simulink model "SiL"  (R2021a)
settings: Solver=VariableStepAuto  StartTime=0.0  StopTime=20  RelTol=1e-3
model workspace: external: MATLAB File C:\Users\Adam\OneDrive\Desktop\M.Sc_LRT\4.sem\session2\Stage\sim\InitMain.m (data not in the file)
values from neighbouring files (symbols this model uses):
  A_mpc = blkdiag([1 dt 0;0 1 dt;0 0 1],[1 dt 0;0 1 dt;0 0 1],[1 dt 0;0 1 dt;0 0 1])    [InitMain.m]    (also in init.m)
  B_mpc = zeros(9,3)    [InitMain.m]    (also in init.m)
  C_mpc = [1 zeros(1,8);0 0 0 1 zeros(1,5); zeros(1,6) 1 0 0 ... (first row only)    [InitMain.m]    (also in init.m)
  D_mpc = zeros(9,3)    [InitMain.m]    (also in init.m)
  dt = 0.01    [InitMain.m]    (also in init.m)
  g0 = 9.81    [InitMain.m]    (also in init.m)
  Ib = diag([0.035 0.046 0.0977])    [InitMain.m]    (also in init.m)
  K1 = Ka(:,1:12)    [InitMain.m]    (also in init.m)
  Ki = -Ka(:,13:16)    [InitMain.m]    (also in init.m)
  M = 1.5    [InitMain.m]    (also in init.m)
  wait = 5    [InitMain.m]    (also in init.m)
undefined symbols (not defined in the file or in its folder): C, Discrete, K_omega, k_omega, Kd_x, Kd_y, Kd_z, Ki_x, Ki_y, Ki_z, Kp_x, Kp_y, Kp_z, Kq_xy, Kq_z, kr, kv, kx, Time
libraries: sharedutil x7, vrlib x5, aerolibutil x3, sharedtransform x2, shared6dof x1, ctrlSharedLib x1, mpclib x1, drivingscenarioandsensors x1
settings Model: Creator=Adam  LastModifiedBy=Adam
settings SolverCC: ZeroCrossAlgorithm=Adaptive
settings DebuggingCC: MaskedZcDiagnostic=none  IgnoredZcDiagnostic=none  UnderSpecifiedDimensionMsg=warning

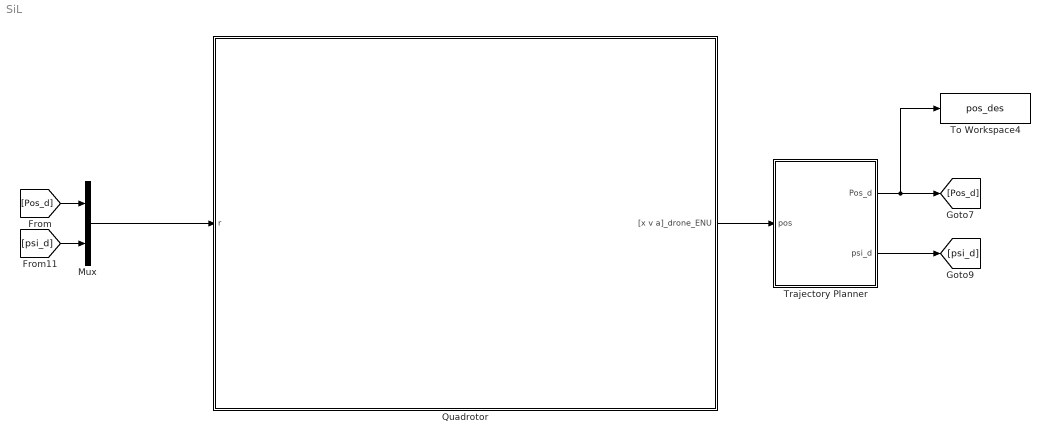
== system SiL ==
  Mux : Mux  Inputs=2
  Quadrotor : Subsystem
      mask Display: image('R.jpg'); % Use "Edit Image" on toolstrip to change.
  To Workspace4 : ToWorkspace  VariableName=pos_des  SaveFormat=Timeseries  SampleTime=-1
  Trajectory Planner : Subsystem
  wires:
  Trajectory Planner/1(Pos_d) -> To Workspace4/1, [Pos_d]
  Trajectory Planner/2(psi_d) -> [psi_d]
  [psi_d] -> Mux/2
  Mux/1 -> Quadrotor/1(r)
  [Pos_d] -> Mux/1
  Quadrotor/1("[x v a]_drone_ENU") -> Trajectory Planner/1(pos)

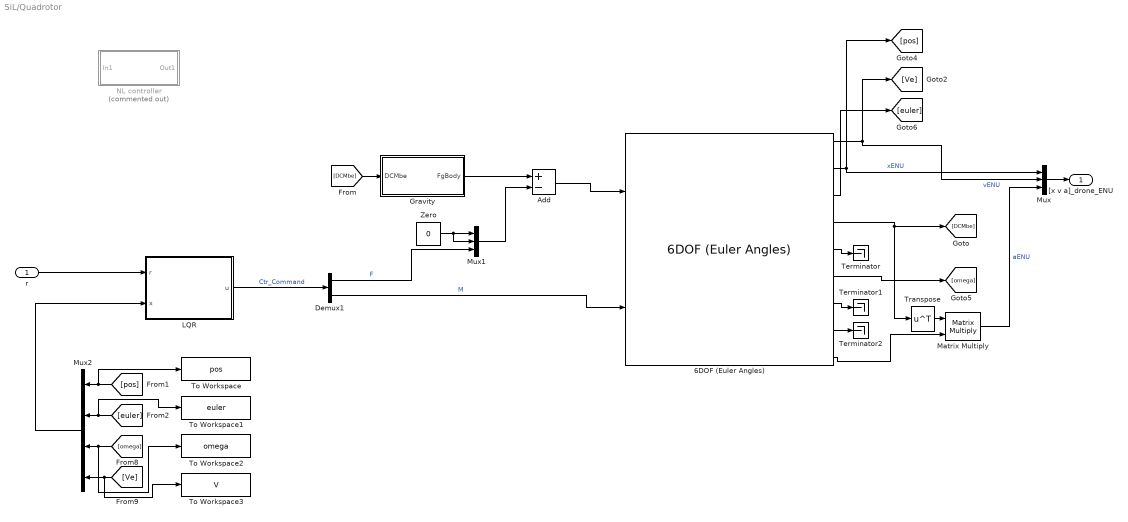
== system SiL/Quadrotor ==
  r : Inport
  6DOF (Euler Angles) : shared6dof/6DOF (Euler Angles)  units=Metric (MKS)  mtype=Fixed  rep=Euler Angles  xme_0=[0 0 0]  Vm_0=[0 0 0]  eul_0=[0 0 0]  pm_0=[0 0 0]  mass_0=M  mass_e=0.5  mass_f=2.0  inertia=Ib  inertia_e=eye(3)  inertia_f=2*eye(3)  k_quat=1.0  vre_flag=on  abi_flag=on  aMode=0  xme_statename='Xe'  Vm_statename='Ve'  eul_statename='Euler'  quat_statename=''  pm_statename='Omega'  mass_statename=''
      settings: SourceProductBaseCode=AE,PW,DR,MT,UV,VE
  Add : Sum  Inputs=+-
  Demux1 : Demux  Outputs=2
  "Gravity " : Subsystem
  LQR : Subsystem
  Matrix Multiply : Product  Multiplication=Matrix(*)
  Mux : Mux  Inputs=3
  Mux1 : Mux  Inputs=3
  Mux2 : Mux
  NL controller : Subsystem  Commented=on
  Terminator : Terminator
  Terminator1 : Terminator
  Terminator2 : Terminator
  To Workspace : ToWorkspace  VariableName=pos  SaveFormat=Timeseries  SampleTime=-1
  To Workspace1 : ToWorkspace  VariableName=euler  SaveFormat=Timeseries  SampleTime=-1
  To Workspace2 : ToWorkspace  VariableName=omega  SaveFormat=Timeseries  SampleTime=-1
  To Workspace3 : ToWorkspace  VariableName=V  SaveFormat=Timeseries  SampleTime=-1
  Transpose : Math  Operator=transpose  SaturateOnIntegerOverflow=on
  Zero : Constant  Value=0  OutDataTypeStr=Inherit: Inherit via back propagation
  "[x v a]_drone_ENU" : Outport
  wires:
  6DOF (Euler Angles)/7 -> Terminator1/1
  "Gravity "/1(FgBody) -> Add/1
  Add/1 -> 6DOF (Euler Angles)/1
  [DCMbe] -> "Gravity "/1(DCMbe)
  6DOF (Euler Angles)/1 -> Mux/2, [Ve]  "vENU"
  6DOF (Euler Angles)/2 -> Mux/1, [pos]  "xENU"
  6DOF (Euler Angles)/3 -> [euler]
  6DOF (Euler Angles)/6 -> [omega]
  6DOF (Euler Angles)/4 -> Transpose/1, [DCMbe]
  Zero/1 -> Mux1/2, Mux1/1
  Mux1/1 -> Add/2
  Demux1/1 -> Mux1/3  "F"
  Demux1/2 -> 6DOF (Euler Angles)/2  "M"
  Mux2/1 -> LQR/2(x)
  [pos] -> To Workspace/1, Mux2/1
  [euler] -> To Workspace1/1, Mux2/2
  LQR/1(u) -> Demux1/1  "Ctr_Command"
  [omega] -> To Workspace2/1, Mux2/3
  [Ve] -> Mux2/4, To Workspace3/1
  r/1 -> LQR/1(r)
  6DOF (Euler Angles)/5 -> Terminator/1
  Transpose/1 -> Matrix Multiply/1
  Matrix Multiply/1 -> Mux/3  "aENU"
  Mux/1 -> "[x v a]_drone_ENU"/1
  6DOF (Euler Angles)/9 -> Matrix Multiply/2
  6DOF (Euler Angles)/8 -> Terminator2/1

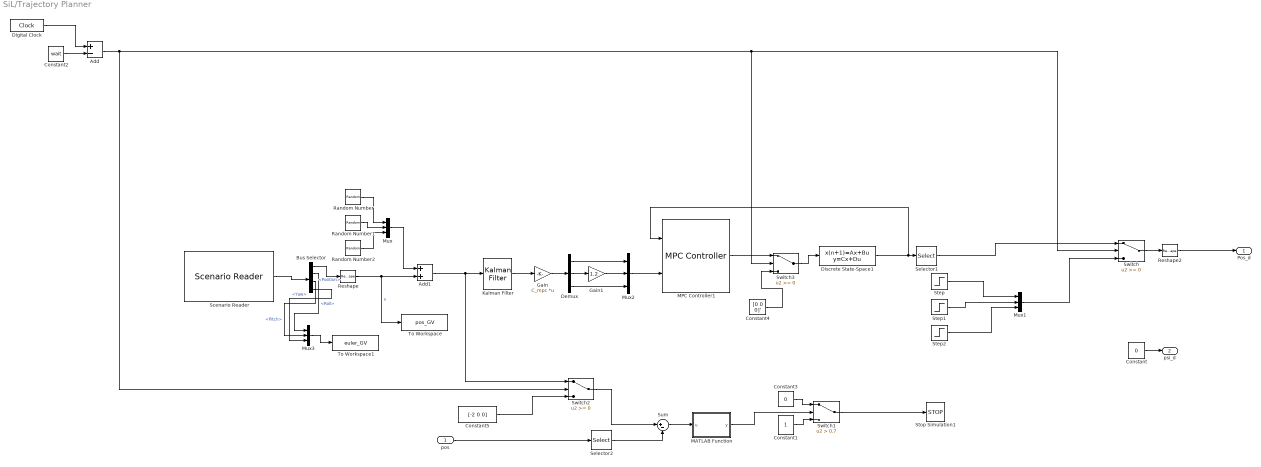
== system SiL/Trajectory Planner ==
  pos : Inport
  Add : Sum  Inputs=+-
  Add1 : Sum
  Bus Selector : BusSelector  OutputSignals=Actors.Position,Actors.Roll,Actors.Pitch,Actors.Yaw
  Constant : Constant  Value=0
  Constant1 : Constant
  Constant2 : Constant  Value=wait
  Constant3 : Constant  Value=0
  Constant4 : Constant  Value=[0 0 0]'
  Constant5 : Constant  Value=[-2 0 0]
  Demux : Demux  Outputs=3
  Digital Clock : DigitalClock  SampleTime=0.01
  Discrete State-Space1 : DiscreteStateSpace  A=A_mpc  B=B_mpc  C=C_mpc  D=D_mpc  InitialCondition="[0;0;0; 0;0;0  ; 5 ;0;0]"  SampleTime=0.01
  Gain : Gain  Gain=C_mpc  Multiplication=Matrix(K*u)
  Gain1 : Gain  Gain=1.2
  Kalman Filter : ctrlSharedLib/Kalman Filter  TimeDomain=Discrete-Time  UseCurrentEstimator=on  ModelSource=Individual A, B, C, D matrices  ModelSourceVariable=ss(0.95,1,1,0,1)  A=blkdiag([1 dt 0.5*dt^2;0 1 dt;0 0 1],[1 dt 0.5*dt^2;0 1 dt;0 0 1],[1 dt 0.5*dt^2;0 1 dt;0 0 1])  B=zeros(  C=[1 zeros(1,8); 0 0 0 1 zeros(1,5); zeros(1,6) 1 0 0]  D=0  NumberOfStates=1  NumberOfInputs=1  NumberOfOutputs=1  InitialEstimateSource=Dialog  X0=zeros(9,1)  P0=10  UseK=off  UseGH=on  NumberOfProcessNoiseInputs=1  G=eye(9)  TimeInvariantG=on  H=0  TimeInvariantH=on  Q=eye(9)*0.01  TimeInvariantQ=on  R=eye(3)*0.01  TimeInvariantR=on  N=0  TimeInvariantN=on  AddInputPort=off  AddEnablePort=off  OutputEstimatedY=off  OutputP=off  Ts=0.01
  MATLAB Function : MATLAB Function  TreatAsAtomicUnit=on
  MPC Controller1 : mpclib/MPC Controller  SCDEnableBlockLinearizationSpecification=on  mpcobj=mpc1  is_multiple=0  enable_value=0  return_u0=off  updateMPCinCallerWorkspace=on  md_inport=off  mv_inport=off  uref_inport=off  return_cost=off  return_mvseq=off  return_qpstatus=off  return_xseq=off  return_state=off  return_ovseq=off  state_inport=off  umin_inport=off  umax_inport=off  ymin_inport=off  ymax_inport=off  cc_inport=off  ywt_inport=off  uwt_inport=off  duwt_inport=off  rhoeps_inport=off  pm_inport=off  MaximumP=10  HorizonChoice=FixedHorizon  n_ts=0.01  n_p=10  n_mv=3  n_md=0  n_ud=0  n_mo=9  n_uo=0  BlockDataType=double  SampleTimeInherited=off  switch_inport=off
  Mux{,1..3} (4 alike) : Mux  Inputs=3
  Random Number : RandomNumber  Variance=0.01  SampleTime=0.01  VectorParams1D=off
  Random Number1 : RandomNumber  Variance=0.01  SampleTime=0.01  VectorParams1D=off
  Random Number2 : RandomNumber  Variance=0.01  SampleTime=0.01  VectorParams1D=off
  Reshape : Reshape
  Reshape2 : Reshape
  Scenario Reader : drivingscenarioandsensors/Scenario Reader  ScenarioSource=From file  ScenarioFileName=C:\Users\Adam\OneDrive\Desktop\M.Sc_LRT\4.sem\session2\Stage\sim\Scenarios\scenario3.mat  ScenarioVariableName=scenario  OutputCoordinateSystem=World coordinates  EgoVehicleSource=Scenario  EgoVehicleActorID=1  OrientVehiclesOnRoad=off  OutputEgoVehiclePose=off  SampleTime=0.01  LaneBoundaryOutput=None  LaneBoundaryDistance=0:0.5:9.5  LaneBoundaryLocation=Center of lane markings  BusNameSource=Auto  BusName=BusActors  BusNumActorsSource=Scenario  BusNumActors=100  BusName2Source=Auto  BusName2=BusLaneBoundaries  BusNumLaneBoundariesSource=Scenario  BusNumLaneBoundaries=10  BusName3Source=Auto  BusName3=BusEgoActor  ShowCoordinateLabels=on  SimulateUsing=Interpreted execution
  Selector1 : Selector  InputPortWidth=9  IndexOptions=Index vector (dialog)  Indices=[1 2 3]  OutputSizes=1
  Selector2 : Selector  InputPortWidth=9  IndexOptions=Index vector (dialog)  Indices=[1 2 3]  OutputSizes=1
  Step : Step  Time=0  After=0  SampleTime=0
  Step1 : Step  Time=0  After=0  SampleTime=0
  Step2 : Step  Time=0  After=5  SampleTime=0
  Stop Simulation1 : Stop
  Sum : Sum  Inputs=|+-
  Switch : Switch
  Switch1 : Switch  Criteria=u2 > Threshold  Threshold=0.7
  Switch2 : Switch
  Switch3 : Switch
  To Workspace : ToWorkspace  VariableName=pos_GV  SaveFormat=Timeseries  SampleTime=-1
  To Workspace1 : ToWorkspace  VariableName=euler_GV  SaveFormat=Timeseries  SampleTime=-1
  Pos_d : Outport
  psi_d : Outport  Port=2
  wires:
  Constant/1 -> psi_d/1
  Step1/1 -> Mux1/2
  Step/1 -> Mux1/1
  Step2/1 -> Mux1/3
  Reshape2/1 -> Pos_d/1
  Discrete State-Space1/1 -> MPC Controller1/1, Selector1/1
  Constant2/1 -> Add/2
  Constant1/1 -> Switch1/3
  MATLAB Function/1(y) -> Switch1/2
  Sum/1 -> MATLAB Function/1(u)
  Switch1/1 -> Stop Simulation1/1
  Constant3/1 -> Switch1/1
  pos/1 -> Selector2/1
  Selector2/1 -> Sum/2
  Digital Clock/1 -> Add/1
  Switch/1 -> Reshape2/1
  Mux1/1 -> Switch/3
  Selector1/1 -> Switch/1
  Switch2/1 -> Sum/1
  Constant5/1 -> Switch2/3
  Add/1 -> Switch2/2, Switch3/2, Switch/2
  Switch3/1 -> Discrete State-Space1/1
  MPC Controller1/1 -> Switch3/1
  Constant4/1 -> Switch3/3
  Add1/1 -> Switch2/1, Kalman Filter/1
  Random Number2/1 -> Mux/3
  Random Number1/1 -> Mux/2
  Reshape/1 -> To Workspace/1, Add1/2  "x"
  Random Number/1 -> Mux/1
  Scenario Reader/1 -> Bus Selector/1
  Bus Selector/1 -> Reshape/1  "<Position>"
  Kalman Filter/1 -> Gain/1
  Mux/1 -> Add1/1
  Gain/1 -> Demux/1
  Demux/2 -> Gain1/1
  Gain1/1 -> Mux2/2
  Demux/1 -> Mux2/1
  Demux/3 -> Mux2/3
  Mux2/1 -> MPC Controller1/2
  Bus Selector/2 -> Mux3/1  "<Roll>"
  Bus Selector/3 -> Mux3/2  "<Pitch>"
  Bus Selector/4 -> Mux3/3  "<Yaw>"
  Mux3/1 -> To Workspace1/1

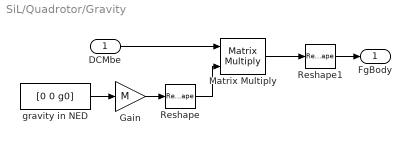
== system SiL/Quadrotor/Gravity  ==
  DCMbe : Inport
  Gain : Gain  Gain=M
  Matrix Multiply : Product  Multiplication=Matrix(*)
  Reshape : Reshape  OutputDimensionality=Column vector (2-D)
  Reshape1 : Reshape
  gravity in NED : Constant  Value=[0 0 g0]
  FgBody : Outport
  wires:
  gravity in NED/1 -> Gain/1
  Reshape/1 -> Matrix Multiply/2
  Matrix Multiply/1 -> Reshape1/1
  DCMbe/1 -> Matrix Multiply/1
  Gain/1 -> Reshape/1
  Reshape1/1 -> FgBody/1

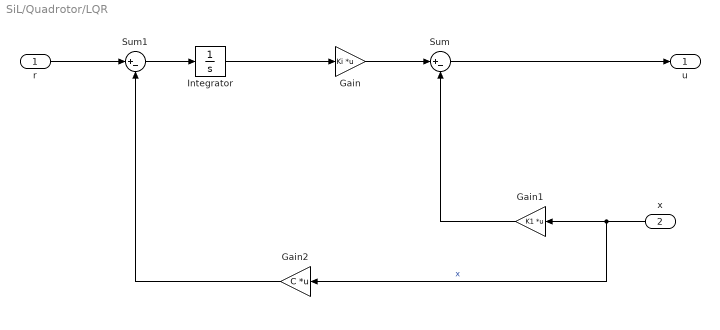
== system SiL/Quadrotor/LQR ==
  r : Inport
  x : Inport  Port=2
  Gain : Gain  Gain=Ki  Multiplication=Matrix(K*u)
  Gain1 : Gain  Gain=K1  Multiplication=Matrix(K*u)
  Gain2 : Gain  Gain=C  Multiplication=Matrix(K*u)
  Integrator : Integrator
  Sum : Sum  Inputs=|+-
  Sum1 : Sum  Inputs=|+-
  u : Outport
  wires:
  Sum/1 -> u/1
  Gain2/1 -> Sum1/2
  r/1 -> Sum1/1
  Gain/1 -> Sum/1
  Sum1/1 -> Integrator/1
  x/1 -> Gain1/1, Gain2/1  "x"
  Gain1/1 -> Sum/2
  Integrator/1 -> Gain/1

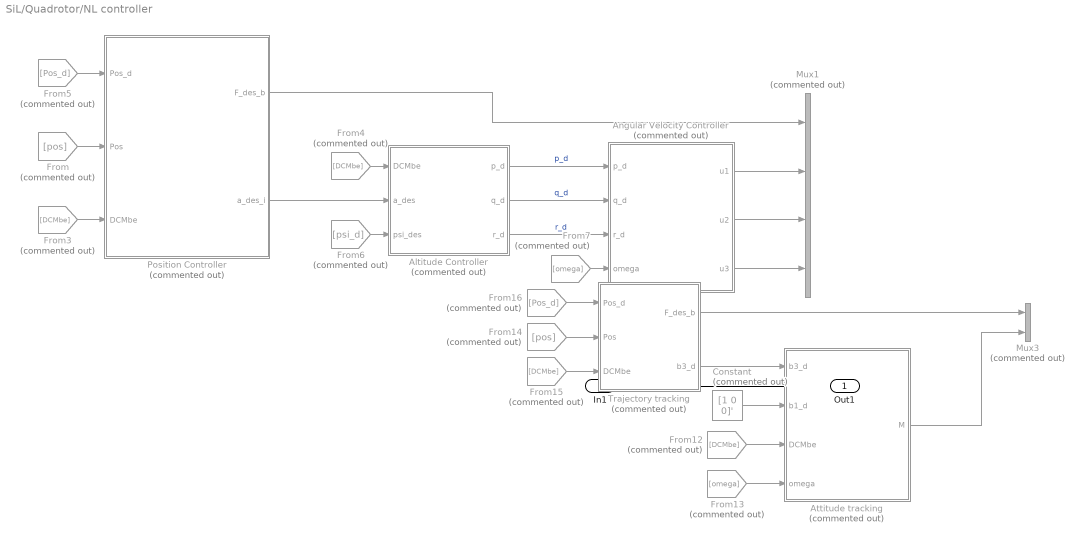
== system SiL/Quadrotor/NL controller ==
  In1 : Inport
  Altitude Controller : Subsystem  Commented=on
  Angular Velocity Controller : Subsystem  Commented=on
  Attitude tracking : Subsystem  Commented=on
  Constant : Constant  Commented=on  Value=[1 0 0]'
  From : From  Commented=on  GotoTag=pos
  From{3..4,12,15} (4 alike) : From  Commented=on  GotoTag=DCMbe
  From13 : From  Commented=on  GotoTag=omega
  From14 : From  Commented=on  GotoTag=pos
  From16 : From  Commented=on  GotoTag=Pos_d
  From5 : From  Commented=on  GotoTag=Pos_d
  From6 : From  Commented=on  GotoTag=psi_d
  From7 : From  Commented=on  GotoTag=omega
  Mux1 : Mux  Commented=on
  Mux3 : Mux  Commented=on  Inputs=2
  Position Controller : Subsystem  Commented=on
  Trajectory tracking : Subsystem  Commented=on
  Out1 : Outport
  wires:
  In1/1 -> Out1/1
  From16/1 -> Trajectory tracking/1(Pos_d)
  Trajectory tracking/1(F_des_b) -> Mux3/1
  From12/1 -> Attitude tracking/3(DCMbe)
  From15/1 -> Trajectory tracking/3(DCMbe)
  From14/1 -> Trajectory tracking/2(Pos)
  Trajectory tracking/2(b3_d) -> Attitude tracking/1(b3_d)
  Constant/1 -> Attitude tracking/2(b1_d)
  From13/1 -> Attitude tracking/4(omega)
  Attitude tracking/1(M) -> Mux3/2
  From7/1 -> Angular Velocity Controller/4(omega)
  Position Controller/1(F_des_b) -> Mux1/1
  From6/1 -> Altitude Controller/3(psi_des)
  Angular Velocity Controller/3(u3) -> Mux1/4
  Altitude Controller/1(p_d) -> Angular Velocity Controller/1(p_d)  "p_d"
  Altitude Controller/3(r_d) -> Angular Velocity Controller/3(r_d)  "r_d"
  Position Controller/2(a_des_i) -> Altitude Controller/2(a_des)
  From/1 -> Position Controller/2(Pos)
  Angular Velocity Controller/1(u1) -> Mux1/2
  From5/1 -> Position Controller/1(Pos_d)
  From3/1 -> Position Controller/3(DCMbe)
  From4/1 -> Altitude Controller/1(DCMbe)
  Altitude Controller/2(q_d) -> Angular Velocity Controller/2(q_d)  "q_d"
  Angular Velocity Controller/2(u2) -> Mux1/3

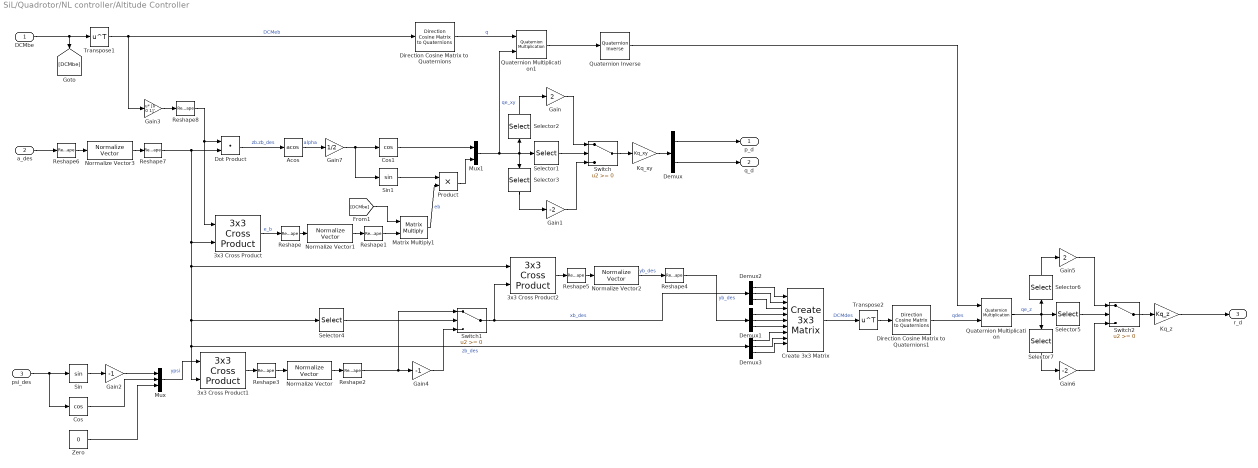
== system SiL/Quadrotor/NL controller/Altitude Controller ==
  DCMbe : Inport
  a_des : Inport  Port=2
  psi_des : Inport  Port=3
  3x3 Cross Product : sharedutil/3x3 Cross Product  aMode=aMode
      settings: SourceProductBaseCode=AE,PW,DR,MT,UV,VE
  3x3 Cross Product1 : sharedutil/3x3 Cross Product  aMode=aMode
      settings: SourceProductBaseCode=AE,PW,DR,MT,UV,VE
  3x3 Cross Product2 : sharedutil/3x3 Cross Product  aMode=aMode
      settings: SourceProductBaseCode=AE,PW,DR,MT,UV,VE
  Acos : Trigonometry  Operator=acos
  Cos : Trigonometry  Operator=cos
  Cos1 : Trigonometry  Operator=cos
  Create 3x3 Matrix : sharedutil/Create 3x3 Matrix  aMode=aMode
      settings: SourceProductBaseCode=AE,PW,DR,MT,UV,VE
  Demux : Demux  Outputs=2
  Demux1 : Demux  Outputs=3
  Demux2 : Demux  Outputs=3
  Demux3 : Demux  Outputs=3
  Direction Cosine Matrix to Quaternions : sharedtransform/Direction Cosine Matrix  to Quaternions  aMode=0  action=None  tolerance=eps(2)
      settings: SourceProductBaseCode=AE,PW,DR,MT,UV,VE
  Direction Cosine Matrix to Quaternions1 : sharedtransform/Direction Cosine Matrix  to Quaternions  aMode=0  action=None  tolerance=eps(2)
      settings: SourceProductBaseCode=AE,PW,DR,MT,UV,VE
  Dot Product : DotProduct  InputSameDT=on  OutDataTypeStr=Inherit: Inherit via internal rule
  Gain : Gain  Gain=2
  Gain1 : Gain  Gain=-2
  Gain2 : Gain  Gain=-1
  Gain3 : Gain  Gain=[0 0 1]'  Multiplication=Matrix(u*K)
  Gain4 : Gain  Gain=-1
  Gain5 : Gain  Gain=2
  Gain6 : Gain  Gain=-2
  Gain7 : Gain  Gain=1/2
  Kq_xy : Gain  Gain=Kq_xy
  Kq_z : Gain  Gain=Kq_z
  Matrix Multiply1 : Product  Multiplication=Matrix(*)
  Mux : Mux  Inputs=3
  Mux1 : Mux  Inputs=2
  Normalize Vector{,1..3} (4 alike) : vrlib/Utilities/Normalize Vector  maxzero=0
  Product : Product
  Quaternion Inverse : aerolibutil/Quaternion Inverse
  Quaternion Multiplication : aerolibutil/Quaternion Multiplication
  Quaternion Multiplication1 : aerolibutil/Quaternion Multiplication
  Reshape{,3,5..6} (4 alike) : Reshape  OutputDimensionality=Column vector (2-D)
  Reshape{1..2,4,7..8} (5 alike) : Reshape
  Selector1 : Selector  InputPortWidth=4  IndexOptions=Index vector (dialog)  Indices=[1 ]  OutputSizes=1
  Selector2 : Selector  InputPortWidth=4  IndexOptions=Index vector (dialog)  Indices=[2 3]  OutputSizes=1
  Selector3 : Selector  InputPortWidth=4  IndexOptions=Index vector (dialog)  Indices=[2 3]  OutputSizes=1
  Selector4 : Selector  InputPortWidth=3  IndexOptions=Index vector (dialog)  Indices=[3]  OutputSizes=1
  Selector5 : Selector  InputPortWidth=4  IndexOptions=Index vector (dialog)  Indices=[1 ]  OutputSizes=1
  Selector6 : Selector  InputPortWidth=4  IndexOptions=Index vector (dialog)  Indices=[4]  OutputSizes=1
  Selector7 : Selector  InputPortWidth=4  IndexOptions=Index vector (dialog)  Indices=[4]  OutputSizes=1
  Sin : Trigonometry
  Sin1 : Trigonometry
  Switch : Switch
  Switch1 : Switch
  Switch2 : Switch
  Transpose1 : Math  Operator=transpose  SaturateOnIntegerOverflow=on
  Transpose2 : Math  Operator=transpose  SaturateOnIntegerOverflow=on
  Zero : Constant  Value=0  OutDataTypeStr=Inherit: Inherit via back propagation
  p_d : Outport
  q_d : Outport  Port=2
  r_d : Outport  Port=3
  wires:
  a_des/1 -> Reshape6/1
  DCMbe/1 -> Transpose1/1, [DCMbe]
  Direction Cosine Matrix to Quaternions/1 -> Quaternion Multiplication1/1  "q"
  Reshape7/1 -> Dot Product/2, 3x3 Cross Product/2, 3x3 Cross Product2/1, Selector4/1, Demux3/1, 3x3 Cross Product1/2  "zb_des"
  Dot Product/1 -> Acos/1  "zb.zb_des"
  Acos/1 -> Gain7/1  "alpha"
  Mux1/1 -> Quaternion Multiplication1/2, Selector1/1, Selector3/1, Selector2/1  "qe_xy"
  Selector1/1 -> Switch/2
  Gain/1 -> Switch/1
  Gain1/1 -> Switch/3
  Switch/1 -> Kq_xy/1
  Kq_xy/1 -> Demux/1
  Selector2/1 -> Gain/1
  Selector3/1 -> Gain1/1
  Zero/1 -> Mux/3
  Mux/1 -> 3x3 Cross Product1/1  "ypsi"
  3x3 Cross Product/1 -> Reshape/1  "e_b"
  Selector4/1 -> Switch1/2
  Gain4/1 -> Switch1/3
  Switch1/1 -> Demux2/1, 3x3 Cross Product2/2  "xb_des"
  Sin/1 -> Gain2/1
  psi_des/1 -> Cos/1, Sin/1
  Gain2/1 -> Mux/1
  Cos/1 -> Mux/2
  Normalize Vector2/1 -> Reshape4/1  "yb_des"
  Create 3x3 Matrix/1 -> Transpose2/1  "DCMdes"
  Direction Cosine Matrix to Quaternions1/1 -> Quaternion Multiplication/2  "qdes"
  Quaternion Multiplication1/1 -> Quaternion Inverse/1
  Quaternion Inverse/1 -> Quaternion Multiplication/1
  Quaternion Multiplication/1 -> Selector7/1, Selector6/1, Selector5/1  "qe_z"
  Gain6/1 -> Switch2/3
  Gain5/1 -> Switch2/1
  Selector5/1 -> Switch2/2
  Selector7/1 -> Gain6/1
  Switch2/1 -> Kq_z/1
  Selector6/1 -> Gain5/1
  Gain3/1 -> Reshape8/1
  Reshape/1 -> Normalize Vector1/1
  Normalize Vector1/1 -> Reshape1/1
  Normalize Vector/1 -> Reshape2/1
  Reshape2/1 -> Switch1/1, Gain4/1
  3x3 Cross Product1/1 -> Reshape3/1
  Reshape3/1 -> Normalize Vector/1
  Reshape4/1 -> Demux1/1  "yb_des"
  3x3 Cross Product2/1 -> Reshape5/1
  Reshape5/1 -> Normalize Vector2/1
  Demux1/1 -> Create 3x3 Matrix/4
  Demux1/2 -> Create 3x3 Matrix/5
  Demux1/3 -> Create 3x3 Matrix/6
  Demux2/1 -> Create 3x3 Matrix/1
  Demux2/2 -> Create 3x3 Matrix/2
  Demux2/3 -> Create 3x3 Matrix/3
  Demux3/1 -> Create 3x3 Matrix/7
  Demux3/2 -> Create 3x3 Matrix/8
  Demux3/3 -> Create 3x3 Matrix/9
  Reshape6/1 -> Normalize Vector3/1
  Normalize Vector3/1 -> Reshape7/1
  Gain7/1 -> Sin1/1, Cos1/1
  Cos1/1 -> Mux1/1
  Product/1 -> Mux1/2
  Demux/1 -> p_d/1
  Demux/2 -> q_d/1
  Kq_z/1 -> r_d/1
  Transpose1/1 -> Direction Cosine Matrix to Quaternions/1, Gain3/1  "DCMeb"
  Transpose2/1 -> Direction Cosine Matrix to Quaternions1/1
  Reshape8/1 -> 3x3 Cross Product/1, Dot Product/1
  Reshape1/1 -> Matrix Multiply1/2
  [DCMbe] -> Matrix Multiply1/1
  Sin1/1 -> Product/1
  Matrix Multiply1/1 -> Product/2  "eb"

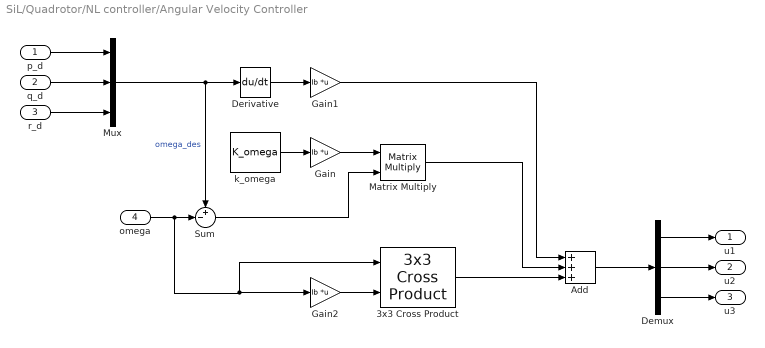
== system SiL/Quadrotor/NL controller/Angular Velocity Controller ==
  p_d : Inport
  q_d : Inport  Port=2
  r_d : Inport  Port=3
  omega : Inport  Port=4
  3x3 Cross Product : sharedutil/3x3 Cross Product  aMode=aMode
      settings: SourceProductBaseCode=AE,PW,DR,MT,UV,VE
  Add : Sum  Inputs=+++
  Demux : Demux  Outputs=3
  Derivative : Derivative
  Gain : Gain  Gain=Ib  Multiplication=Matrix(K*u)
  Gain1 : Gain  Gain=Ib  Multiplication=Matrix(K*u)
  Gain2 : Gain  Gain=Ib  Multiplication=Matrix(K*u)
  Matrix Multiply : Product  Multiplication=Matrix(*)
  Mux : Mux  Inputs=3
  Sum : Sum  Inputs=+-|
  k_omega : Constant  Value=K_omega
  u1 : Outport
  u2 : Outport  Port=2
  u3 : Outport  Port=3
  wires:
  k_omega/1 -> Gain/1
  Gain/1 -> Matrix Multiply/1
  Sum/1 -> Matrix Multiply/2
  omega/1 -> Gain2/1, 3x3 Cross Product/1, Sum/2
  Gain2/1 -> 3x3 Cross Product/2
  Derivative/1 -> Gain1/1
  3x3 Cross Product/1 -> Add/3
  Matrix Multiply/1 -> Add/2
  Gain1/1 -> Add/1
  Add/1 -> Demux/1
  Demux/1 -> u1/1
  Demux/2 -> u2/1
  Demux/3 -> u3/1
  Mux/1 -> Sum/1, Derivative/1  "omega_des"
  p_d/1 -> Mux/1
  q_d/1 -> Mux/2
  r_d/1 -> Mux/3

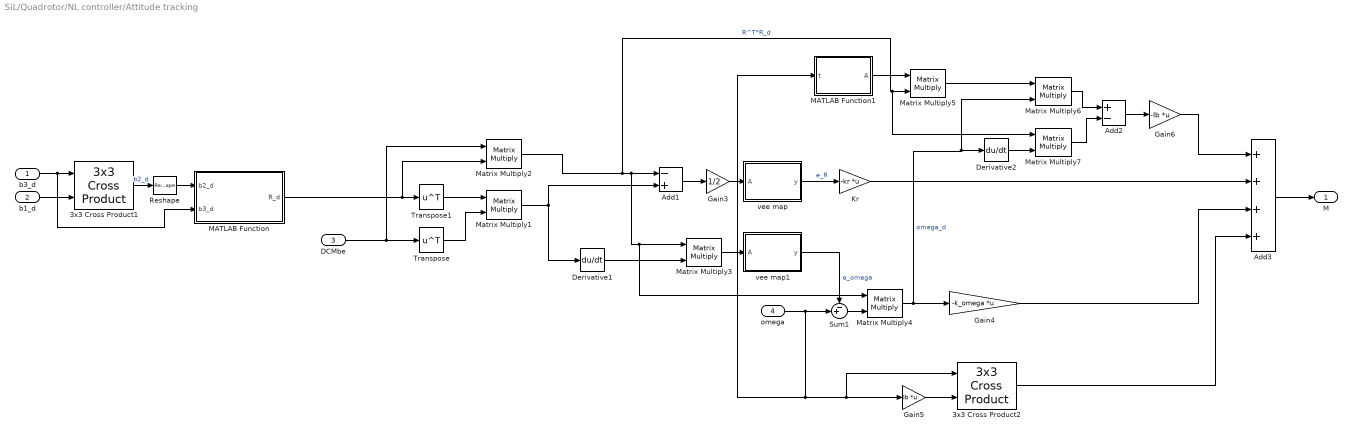
== system SiL/Quadrotor/NL controller/Attitude tracking ==
  b3_d : Inport
  b1_d : Inport  Port=2
  DCMbe : Inport  Port=3
  omega : Inport  Port=4
  3x3 Cross Product1 : sharedutil/3x3 Cross Product  aMode=aMode
      settings: SourceProductBaseCode=AE,PW,DR,MT,UV,VE
  3x3 Cross Product2 : sharedutil/3x3 Cross Product  aMode=aMode
      settings: SourceProductBaseCode=AE,PW,DR,MT,UV,VE
  Add1 : Sum  Inputs=-+
  Add2 : Sum  Inputs=+-
  Add3 : Sum  Inputs=++++
  Derivative1 : Derivative
  Derivative2 : Derivative
  Gain3 : Gain  Gain=1/2
  Gain4 : Gain  Gain=-k_omega  Multiplication=Matrix(K*u)
  Gain5 : Gain  Gain=Ib  Multiplication=Matrix(K*u)
  Gain6 : Gain  Gain=-Ib  Multiplication=Matrix(K*u)
  Kr : Gain  Gain=-kr  Multiplication=Matrix(K*u)
  MATLAB Function : MATLAB Function  TreatAsAtomicUnit=on
  MATLAB Function1 : MATLAB Function  TreatAsAtomicUnit=on
  Matrix Multiply{1..7} (7 alike) : Product  Multiplication=Matrix(*)
  Reshape : Reshape  OutputDimensionality=Column vector (2-D)
  Sum1 : Sum  Inputs=-+|
  Transpose : Math  Operator=transpose  SaturateOnIntegerOverflow=on
  Transpose1 : Math  Operator=transpose  SaturateOnIntegerOverflow=on
  vee map : MATLAB Function  TreatAsAtomicUnit=on
  vee map1 : MATLAB Function  TreatAsAtomicUnit=on
  M : Outport
  wires:
  b3_d/1 -> MATLAB Function/2(b3_d), 3x3 Cross Product1/1
  b1_d/1 -> 3x3 Cross Product1/2
  DCMbe/1 -> Matrix Multiply2/1, Transpose/1
  MATLAB Function/1(R_d) -> Matrix Multiply2/2, Transpose1/1
  Transpose1/1 -> Matrix Multiply1/1
  Transpose/1 -> Matrix Multiply1/2
  Matrix Multiply2/1 -> Matrix Multiply7/1, Matrix Multiply5/2, Matrix Multiply4/1, Matrix Multiply3/1, Add1/1  "R^T*R_d"
  Add1/1 -> Gain3/1
  Gain3/1 -> vee map/1(A)
  vee map/1(y) -> Kr/1  "e_R"
  Derivative1/1 -> Matrix Multiply3/2
  Matrix Multiply3/1 -> vee map1/1(A)
  vee map1/1(y) -> Sum1/1  "e_omega"
  Sum1/1 -> Matrix Multiply4/2
  Matrix Multiply1/1 -> Derivative1/1, Add1/2
  Matrix Multiply4/1 -> Gain4/1, Derivative2/1, Matrix Multiply6/2  "omega_d"
  omega/1 -> MATLAB Function1/1(t), Gain5/1, 3x3 Cross Product2/1, Sum1/2
  Gain5/1 -> 3x3 Cross Product2/2
  MATLAB Function1/1(A) -> Matrix Multiply5/1
  Matrix Multiply5/1 -> Matrix Multiply6/1
  Derivative2/1 -> Matrix Multiply7/2
  Matrix Multiply6/1 -> Add2/1
  Matrix Multiply7/1 -> Add2/2
  Add2/1 -> Gain6/1
  Gain6/1 -> Add3/1
  Kr/1 -> Add3/2
  Gain4/1 -> Add3/3
  3x3 Cross Product2/1 -> Add3/4
  Add3/1 -> M/1
  3x3 Cross Product1/1 -> Reshape/1  "b2_d"
  Reshape/1 -> MATLAB Function/1(b2_d)

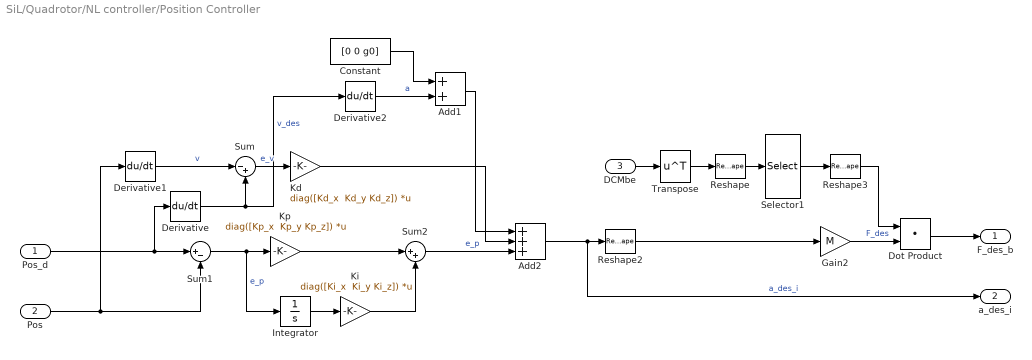
== system SiL/Quadrotor/NL controller/Position Controller ==
  Pos_d : Inport
  Pos : Inport  Port=2
  DCMbe : Inport  Port=3
  Add1 : Sum
  Add2 : Sum  Inputs=+++
  Constant : Constant  Value=[0 0 g0]
  Derivative : Derivative
  Derivative1 : Derivative
  Derivative2 : Derivative
  Dot Product : DotProduct  InputSameDT=on  OutDataTypeStr=Inherit: Inherit via internal rule
  Gain2 : Gain  Gain=M
  Integrator : Integrator
  Kd : Gain  Gain="diag([Kd_x  Kd_y Kd_z])"  Multiplication=Matrix(K*u)
  Ki : Gain  Gain="diag([Ki_x  Ki_y Ki_z])"  Multiplication=Matrix(K*u)
  Kp : Gain  Gain="diag([Kp_x  Kp_y Kp_z])"  Multiplication=Matrix(K*u)
  Reshape : Reshape  OutputDimensionality=Column vector (2-D)
  Reshape2 : Reshape  OutputDimensionality=Column vector (2-D)
  Reshape3 : Reshape
  Selector1 : Selector  InputPortWidth=9  IndexOptions=Index vector (dialog)  Indices=[7 8 9]  OutputSizes=1
  Sum : Sum  Inputs=|-+
  Sum1 : Sum  Inputs=|+-
  Sum2 : Sum  Inputs=|++
  Transpose : Math  Operator=transpose  SaturateOnIntegerOverflow=on
  F_des_b : Outport
  a_des_i : Outport  Port=2
  wires:
  Pos_d/1 -> Sum1/1, Derivative/1
  Pos/1 -> Derivative1/1, Sum1/2
  Sum1/1 -> Integrator/1, Kp/1  "e_p"
  Derivative/1 -> Derivative2/1, Sum/2  "v_des"
  Sum/1 -> Kd/1  "e_v"
  Kd/1 -> Add2/2
  Add2/1 -> a_des_i/1, Reshape2/1  "a_des_i"
  Derivative1/1 -> Sum/1  "v"
  Derivative2/1 -> Add1/2  "a"
  DCMbe/1 -> Transpose/1
  Dot Product/1 -> F_des_b/1
  Gain2/1 -> Dot Product/2  "F_des"
  Integrator/1 -> Ki/1
  Kp/1 -> Sum2/1
  Ki/1 -> Sum2/2
  Sum2/1 -> Add2/3  "e_p"
  Constant/1 -> Add1/1
  Add1/1 -> Add2/1
  Transpose/1 -> Reshape/1
  Reshape/1 -> Selector1/1
  Selector1/1 -> Reshape3/1
  Reshape3/1 -> Dot Product/1
  Reshape2/1 -> Gain2/1

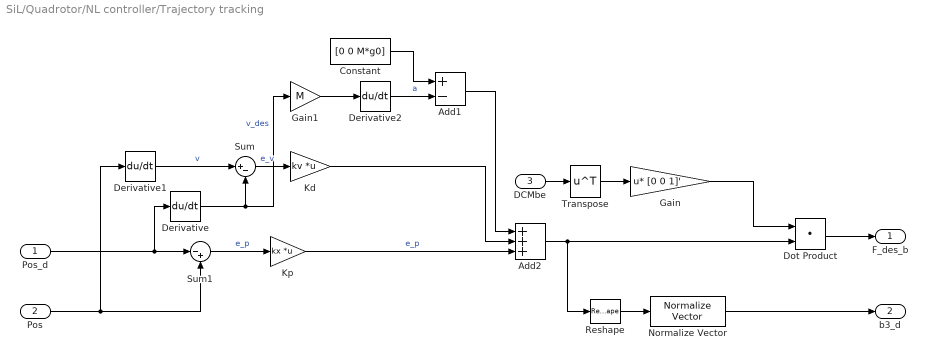
== system SiL/Quadrotor/NL controller/Trajectory tracking ==
  Pos_d : Inport
  Pos : Inport  Port=2
  DCMbe : Inport  Port=3
  Add1 : Sum  Inputs=+-
  Add2 : Sum  Inputs=+++
  Constant : Constant  Value=[0 0 M*g0]
  Derivative : Derivative
  Derivative1 : Derivative
  Derivative2 : Derivative
  Dot Product : DotProduct  InputSameDT=on  OutDataTypeStr=Inherit: Inherit via internal rule
  Gain : Gain  Gain=[0 0 1]'  Multiplication=Matrix(u*K)
  Gain1 : Gain  Gain=M
  Kd : Gain  Gain=kv  Multiplication=Matrix(K*u)
  Kp : Gain  Gain=kx  Multiplication=Matrix(K*u)
  Normalize Vector : vrlib/Utilities/Normalize Vector  maxzero=0
  Reshape : Reshape  OutputDimensionality=Column vector (2-D)
  Sum : Sum  Inputs=|+-
  Sum1 : Sum  Inputs=|-+
  Transpose : Math  Operator=transpose  SaturateOnIntegerOverflow=on
  F_des_b : Outport
  b3_d : Outport  Port=2
  wires:
  Derivative/1 -> Gain1/1, Sum/2  "v_des"
  Derivative1/1 -> Sum/1  "v"
  Kp/1 -> Add2/3  "e_p"
  Derivative2/1 -> Add1/2  "a"
  Add1/1 -> Add2/1
  Transpose/1 -> Gain/1
  Constant/1 -> Add1/1
  Kd/1 -> Add2/2
  Pos_d/1 -> Sum1/1, Derivative/1
  Sum/1 -> Kd/1  "e_v"
  DCMbe/1 -> Transpose/1
  Dot Product/1 -> F_des_b/1
  Add2/1 -> Reshape/1, Dot Product/2
  Pos/1 -> Derivative1/1, Sum1/2
  Sum1/1 -> Kp/1  "e_p"
  Gain1/1 -> Derivative2/1
  Gain/1 -> Dot Product/1
  Reshape/1 -> Normalize Vector/1
  Normalize Vector/1 -> b3_d/1

== matlab function SiL/Quadrotor/NL controller/Attitude tracking/MATLAB Function ==
  data: b2_d input; R_d output; b3_d input
function R_d = Creatematrix(b2_d,b3_d)

R_d = [cross(b2_d,b3_d)'; b2_d' ;b3_d']';

== matlab function SiL/Quadrotor/NL controller/Attitude tracking/vee map1 ==
  data: A input; y output
function y = vee(A)

y = [A(3,2) ;
         A(1,3) ;
         A(2,1)] ;

== matlab function SiL/Quadrotor/NL controller/Attitude tracking/MATLAB Function1 ==
  data: t input; A output
function A = vectorX(t)

A = [0 -t(3) t(2) ; t(3) 0 -t(1) ; -t(2) t(1) 0] ;

== matlab function SiL/Trajectory Planner/MATLAB Function ==
  data: u input; y output
function y = fcn(u)

y = norm(u);

== matlab function SiL/Quadrotor/NL controller/Attitude tracking/vee map ==
  data: A input; y output
function y = vee(A)

y = [A(3,2) ;
         A(1,3) ;
         A(2,1)] ;
